simulink model "mysvm_NLC"  (R2017b)
settings: Solver=ode45  StartTime=0.0  StopTime=0.02  RelTol=1e-3  EnableMultiTasking=on
values from neighbouring files (symbols this model uses):
  N = nlcinput(4) - 1    [MLNLC_m.m]    (also in MLPDPWM_m.m = pdpwminput(4) - 1; MLSVC_m.m = svcinput(4) - 1)
undefined symbols (not defined in the file or in its folder): m
libraries: powerlib x8, powerlib_meascontrol x4
settings Model: Creator=吴鸿达  LastModifiedBy=AdamWu
settings DataIOCC: LimitDataPoints=on  SaveFormat=Array
settings OptimizationCC: LifeSpan=inf
settings DebuggingCC: SolverPrmCheckMsg=warning  UnconnectedInputMsg=none  UnconnectedOutputMsg=none  UnconnectedLineMsg=none  SFUnexpectedBacktrackingDiag=warning  SFNoUnconditionalDefaultTransitionDiag=warning  SFExecutionAtInitializationDiag=none
settings HardwareCC: ProdBitPerPointer=32  ProdBitPerSizeT=32  ProdBitPerPtrDiffT=32  ProdLargestAtomicFloat=None  ProdIntDivRoundTo=Undefined  ProdEndianess=Unspecified  ProdWordSize=32  ProdHWDeviceType=32-bit Generic
settings ModelReferenceCC: PropagateSignalLabelsOutOfModel=off
settings CodeAppCC: StateflowObjectComments=on
settings GRTTargetCC: TargetLangStandard=C89/C90 (ANSI)  GeneratePreprocessorConditionals=Disable all
settings ConfigComp: CovMetricSettings=dw  CovHtmlReporting=on  CovSaveCumulativeToWorkspaceVar=on  CovSaveSingleToWorkspaceVar=on  CovExternalEMLEnable=off  CovSFcnEnable=off
settings SimscapeCC: SimscapeNormalizeSystem=off

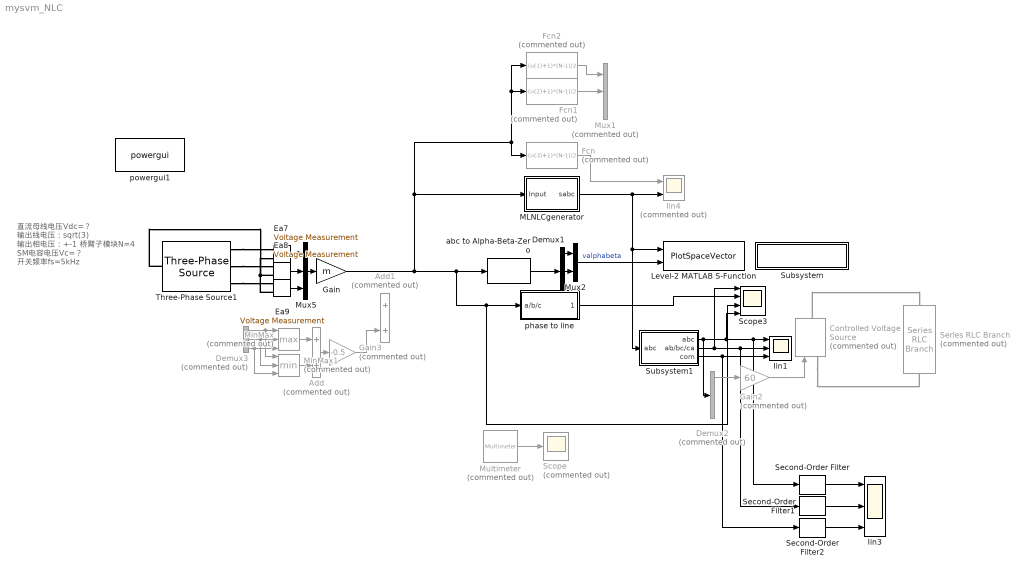
== system mysvm_NLC ==
  note: 直流母线电压Vdc=？
      |
      | 输出线电压：sqrt(3)
      | 输出相电压：+-1
      | 桥臂子模块N=4
      | SM电容电压Vc=？
      | 开关频率fs=5kHz
  Add : Sum  Commented=on
  Add1 : Sum  Commented=on
  Controlled Voltage Source : powerlib/Electrical Sources/Controlled Voltage Source  Commented=on  Initialize=on  Source_Type=AC  Amplitude=0  Phase=0  Frequency=0  Measurements=None
  Demux1 : Demux  Outputs=3
  Demux2 : Demux  Commented=on  Outputs=3
  Demux3 : Demux  Commented=on  Outputs=3
  Ea7 : powerlib/Measurements/Voltage Measurement  PhasorSimulation=off  OutputType=Complex  PSBequivalent=0
  Ea8 : powerlib/Measurements/Voltage Measurement  PhasorSimulation=off  OutputType=Complex  PSBequivalent=0
  Ea9 : powerlib/Measurements/Voltage Measurement  PhasorSimulation=off  OutputType=Complex  PSBequivalent=0
  Fcn : Fcn  Commented=on  Expr=(u(3)+1)*(N-1)/2
  Fcn1 : Fcn  Commented=on  Expr=(u(2)+1)*(N-1)/2
  Fcn2 : Fcn  Commented=on  Expr=(u(1)+1)*(N-1)/2
  Gain : Gain  Gain=m
  Gain2 : Gain  Commented=on  Gain=60
  Gain3 : Gain  Commented=on  Gain=-0.5
  Iin1 : Scope  NumInputPorts=3
  Iin3 : Scope  NumInputPorts=3
  Iin4 : Scope  Commented=on  NumInputPorts=2
  Level-2 MATLAB S-Function : M-S-Function  FunctionName=PlotSpaceVector  Parameters=level, vdc, rate, normalized, plot, hexagon, sw, disabled  mask{disabled=on, level=N, rate=50, vdc=2/50, normalized=on, plot=4, hexagon=off, sw=on}
      mask prompts: disabled "Disable Plot"; level "Voltage Level"; rate "Plot Rate"; vdc "DC Link Voltage"; plot "Plot Number"; sw "Show Switching"
  MLNLCgenerator : Subsystem  mask{level=N, fs=10e3, mode_nlc=off, line_nlc=off}
      mask prompts: level "Voltage Level"; fs "Frequency"; mode_nlc "PWM Mode"; line_nlc "Line-to-line Voltage Mode"
  MinMax : MinMax  Commented=on  Function=max  Inputs=3
  MinMax1 : MinMax  Commented=on  Inputs=3
  Multimeter : powerlib/Measurements/Multimeter  Commented=on  PhasorSimulation=off  OutputType=Complex  sel=[1 2]  L=2  Gain=[1 1]  yselected={'Ub: Series RLC Branch','Ib: Series RLC Branch'};  PSBOutputType=1  PSBequivalent=0  AxesSetting=[0,0.1,-100,100]  Display=1  SavedBlockNames=-11
  Mux1 : Mux  Commented=on  Inputs=3
  Mux2 : Mux  Inputs=2
  Mux5 : Mux  Inputs=3
  Scope : Scope  Commented=on
  Scope3 : Scope  NumInputPorts=4
  Second-Order Filter : powerlib_meascontrol/Filters/Second-Order Filter  FilterType=Lowpass  Fo=1000  Zeta=0.707  Ts=0  Initialize=on  Vac_Init="[0,  0,  50]"  Vdc_Init=0  PlotResponse=off  FreqRange=[0, 500, 1]
      settings: SourceProductName=Simscape Power Systems  SourceProductBaseCode=PS
  Second-Order Filter1 : powerlib_meascontrol/Filters/Second-Order Filter  FilterType=Lowpass  Fo=1000  Zeta=0.707  Ts=0  Initialize=on  Vac_Init="[0,  0,  50]"  Vdc_Init=0.5  PlotResponse=off  FreqRange=[0, 500, 1]
      settings: SourceProductName=Simscape Power Systems  SourceProductBaseCode=PS
  Second-Order Filter2 : powerlib_meascontrol/Filters/Second-Order Filter  FilterType=Lowpass  Fo=1000  Zeta=0.707  Ts=0  Initialize=on  Vac_Init="[0,  0,  50]"  Vdc_Init=0.5  PlotResponse=off  FreqRange=[0, 500, 1]
      settings: SourceProductName=Simscape Power Systems  SourceProductBaseCode=PS
  Series RLC Branch : powerlib/Elements/Series RLC Branch  Commented=on  LConnTagsString=__new0  RConnTagsString=__new0  BranchType=RL  Resistance=80  Inductance=30e-3  SetiL0=off  InitialCurrent=0  Capacitance=1e-6  Setx0=off  InitialVoltage=0  Measurements=Branch voltage and current
  Subsystem : Subsystem  mask{filename=SVPWM_sFunction.m}
      settings: AttributesFormatString=\n  OpenFcn=open('F:\研究生\matlab\PlotSpaceVector.m')
      mask Display:
      | patch([0 1 1 0], [0 0 1 1],[0.2 0.6 0.9])
      | disp('plotspacevector.m')
  Subsystem1 : Subsystem  mask{N=N, normal=on}
      mask prompts: N "Voltage Level"; normal "Normalized"
  Three-Phase Source1 : powerlib/Electrical Sources/Three-Phase Source  InternalConnection=Yn  VoltagePhases=off  Voltage=sqrt(3/2)  PhaseAngle=0.1  Voltage_phases=[25e3 25e3 25e3]/sqrt(3)  PhaseAngles_phases=[0 -120 +120]  Frequency=50  NonIdealSource=off  SpecifyImpedance=off  Resistance=0.8929  Inductance=1e-3  ShortCircuitLevel=100e6  BaseVoltage=25e3  XRratio=7  BusType=swing  Pref=10e3  Qref=0  Prefabc=[10e3, 10e3, 10e3]  Qrefabc=[0, 0, 0]  Qmin=-inf  Qmax=inf
  abc to Alpha-Beta-Zero : powerlib_meascontrol/Transformations/abc to Alpha-Beta-Zero
      settings: SourceProductName=Simscape Power Systems
  phase to line : Subsystem
  powergui1 : powerlib/powergui  Priority=1  SimulationMode=Discrete  SampleTime=0.5e-6  frequency=60  Iterations=50  frequencyindice=50  Pbase=100e6  ErrMax=1e-4  UnitsV=kV  UnitsW=MW  buscounter=0  FunctionMessages=off  echomessages=off  EnableUseOfTLC=off  CurrentSourceSwitches=off  DisableSnubberDevices=off  DisableRonSwitches=off  DisableVfSwitches=off  DisplayEquations=off  SolverType=Tustin/Backward Euler (TBE)  Interpol=off  ExternalGateDelay=off  methode=off  Ts=100  x0status=blocks  SPID=on  SwTol=0  HookPort=off  RestoreLinks=warning  ResistiveCurrentMeasurement=off  Frange=[0:2:500]  Ylog=off  Xlog=on  ShowGrid=off  save=off  variable=ZData  structure=NLCoutput  ZoomFFT=off  StartTime=0.000  cycles=1  DisplayStyle=1  fundamental=50  FreqAxis=on  MaxFrequency=5000  frequencyindicesteady=1  RmsSteady=1  display=off
  wires:
  Ea9/1 -> Mux5/3
  Ea7/1 -> Mux5/1
  Ea8/1 -> Mux5/2
  abc to Alpha-Beta-Zero/1 -> Demux1/1
  Demux1/1 -> Mux2/1
  Demux1/2 -> Mux2/2
  Mux2/1 -> Level-2 MATLAB S-Function/2  "valphabeta"
  Subsystem1/3(com) -> Second-Order Filter2/1, Iin1/3
  MLNLCgenerator/1(sabc) -> Level-2 MATLAB S-Function/1, Subsystem1/1("abc "), Iin4/2
  Fcn/1 -> Iin4/1
  Fcn1/1 -> Mux1/2
  Fcn2/1 -> Mux1/1
  Gain/1 -> MLNLCgenerator/1(Input), Fcn2/1, Fcn1/1, Fcn/1, Scope3/3, phase to line/1(a/b/c), abc to Alpha-Beta-Zero/1
  Demux2/1 -> Gain2/1
  Gain2/1 -> Controlled Voltage Source/1
  Multimeter/1 -> Scope/1
  Second-Order Filter1/1 -> Iin3/2
  Second-Order Filter/1 -> Iin3/1
  Subsystem1/1(abc) -> Demux2/1, Scope3/4, Second-Order Filter/1, Iin1/1
  Subsystem1/2(ab/bc/ca) -> Scope3/1, Iin1/2, Second-Order Filter1/1
  MinMax/1 -> Add/1
  Mux5/1 -> Gain/1
  Add/1 -> Gain3/1
  MinMax1/1 -> Add/2
  Demux3/1 -> MinMax1/1, MinMax/1
  Demux3/2 -> MinMax1/2, MinMax/2
  Demux3/3 -> MinMax1/3, MinMax/3
  Gain3/1 -> Add1/2
  Second-Order Filter2/1 -> Iin3/3
  phase to line/1(ab/bc/ca) -> Scope3/2
  connections:
  Ea9/LConn2 -- Three-Phase Source1/LConn1 -- Ea7/LConn2 -- Ea8/LConn2
  Three-Phase Source1/RConn1 -- Ea7/LConn1
  Three-Phase Source1/RConn2 -- Ea8/LConn1
  Three-Phase Source1/RConn3 -- Ea9/LConn1
  Controlled Voltage Source/RConn1 -- Series RLC Branch/LConn1
  Controlled Voltage Source/LConn1 -- Series RLC Branch/RConn1

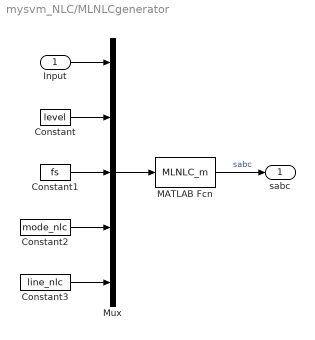
== system mysvm_NLC/MLNLCgenerator ==
  Input : Inport
  Constant : Constant  Value=level
  Constant1 : Constant  Value=fs
  Constant2 : Constant  Value=mode_nlc
  Constant3 : Constant  Value=line_nlc
  MATLAB Fcn : MATLABFcn  MATLABFcn=MLNLC_m  OutputSignalType=real
  Mux : Mux  Inputs=5
  sabc : Outport
  wires:
  MATLAB Fcn/1 -> sabc/1  "sabc"
  Input/1 -> Mux/1
  Constant/1 -> Mux/2
  Mux/1 -> MATLAB Fcn/1
  Constant1/1 -> Mux/3
  Constant2/1 -> Mux/4
  Constant3/1 -> Mux/5

== system mysvm_NLC/Subsystem ==

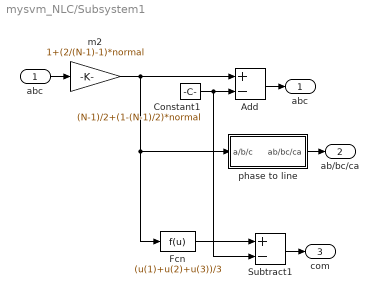
== system mysvm_NLC/Subsystem1 ==
  "abc " : Inport
  Add : Sum  Inputs=+-
  Constant1 : Constant  Value=(N-1)/2+(1-(N-1)/2)*normal
  Fcn : Fcn  Expr=(u(1)+u(2)+u(3))/3
  Subtract1 : Sum  Inputs=+-
  m2 : Gain  Gain=1+(2/(N-1)-1)*normal
  phase to line : Subsystem
  abc : Outport
  ab/bc/ca : Outport  Port=2
  com : Outport  Port=3
  wires:
  Subtract1/1 -> com/1
  "abc "/1 -> m2/1
  Fcn/1 -> Subtract1/1
  Constant1/1 -> Subtract1/2, Add/2
  m2/1 -> Add/1, phase to line/1(a/b/c), Fcn/1
  Add/1 -> abc/1
  phase to line/1(ab/bc/ca) -> ab/bc/ca/1

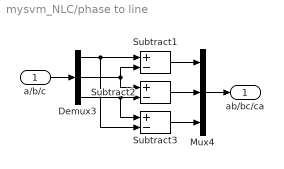
== system mysvm_NLC/phase to line ==
  a/b/c : Inport
  Demux3 : Demux  Outputs=3
  Mux4 : Mux  Inputs=3
  Subtract1 : Sum  Inputs=+-
  Subtract2 : Sum  Inputs=+-
  Subtract3 : Sum  Inputs=+-
  ab/bc/ca : Outport
  wires:
  Subtract2/1 -> Mux4/2
  Subtract1/1 -> Mux4/1
  Demux3/2 -> Subtract2/1, Subtract1/2
  a/b/c/1 -> Demux3/1
  Mux4/1 -> ab/bc/ca/1
  Demux3/3 -> Subtract2/2, Subtract3/1
  Subtract3/1 -> Mux4/3
  Demux3/1 -> Subtract1/1, Subtract3/2

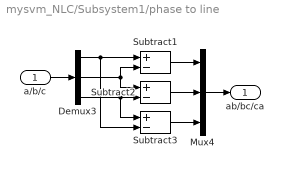
== system mysvm_NLC/Subsystem1/phase to line ==
  a/b/c : Inport
  Demux3 : Demux  Outputs=3
  Mux4 : Mux  Inputs=3
  Subtract1 : Sum  Inputs=+-
  Subtract2 : Sum  Inputs=+-
  Subtract3 : Sum  Inputs=+-
  ab/bc/ca : Outport
  wires:
  Subtract2/1 -> Mux4/2
  Subtract1/1 -> Mux4/1
  Demux3/2 -> Subtract2/1, Subtract1/2
  a/b/c/1 -> Demux3/1
  Mux4/1 -> ab/bc/ca/1
  Demux3/3 -> Subtract2/2, Subtract3/1
  Subtract3/1 -> Mux4/3
  Demux3/1 -> Subtract1/1, Subtract3/2
